simulink model "LinearizationHarness"  (R2017b)
settings: configuration reference "ControlDesignConfigSet" (kept outside this file)
settings Model: Creator=eh6qym  LastModifiedBy=eh6qym
settings ConfigSetRef: SourceLocation=Base Workspace

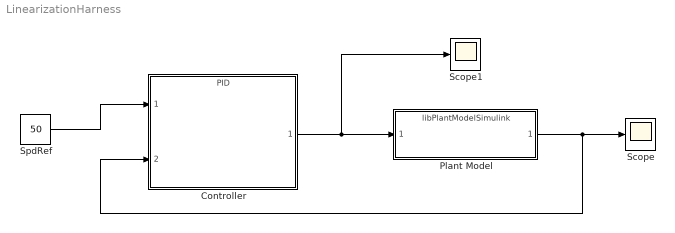
== system LinearizationHarness ==
  Controller : ModelReference  ModelNameDialog=PID.slx  SimulationMode=Normal  ModelReferenceVersion=1.6
  Plant Model : ModelReference  ModelNameDialog=libPlantModelSimulink.mdl  SimulationMode=Normal  ModelReferenceVersion=1.21
  Scope : Scope
  Scope1 : Scope
  SpdRef : Constant  Value=50
  wires:
  Controller/1 -> Scope1/1, Plant Model/1
  Plant Model/1 -> Controller/2, Scope/1
  SpdRef/1 -> Controller/1
